simulink model "check_GearSelector"  (R2018b)
settings: configuration reference "Physics" (kept outside this file)
model workspace (MAT data in the model file):
  veh_param = Simulink.Parameter
  veh_param.Value.cLiftF = 0
  veh_param.Value.cLiftR = 0
  veh_param.Value.CoGx_m = 0
  veh_param.Value.CoGy_m = 0
  veh_param.Value.CoGz_m = 0
  veh_param.Value.cDrag = 0
  veh_param.Value.Aref_m2 = 0
  veh_param.Value.Gearratio = 0
  veh_param.Value.Wheelbase_m = 0
  veh_param.Value.PacLatF = [0 0 0 0 0]
  veh_param.Value.PacLongF = [0 0 0 0 0]
  veh_param.Value.PacLatR = [0 0 0 0 0]
  veh_param.Value.PacLongR = [0 0 0 0 0]
  veh_param.Value.cRollFriction_Npmps = 0
  veh_param.Value.MaxRollFriction_N = 0
  veh_param.Value.T_YawRate_s = 0
  veh_param.Value.T_LatVel_s = 0
  veh_param.Value.TrackWidthF_m = 0
  veh_param.Value.TrackWidthR_m = 0
  veh_param.Value.TireRadiusF_m = 0
  veh_param.Value.TireRadiusR_m = 0
  veh_param.Value.VehicleInertia_kgm2 = 0
  veh_param.Value.WheelInertiaF_kgm2 = 0
  veh_param.Value.WheelInertiaR_kgm2 = 0
  veh_param.Value.VehicleMass_kg = 0
  veh_param.Value.switchModelBlend_mps = 0
  veh_param.Value.PTLimitLowVel_N = 0
  veh_param.Value.switchModelVel_mps = 0
  veh_param.Value.T_Tire_s = 0
  veh_param.DataType = 'struct'
  veh_param.Dimensions = [1 1]
  x0_positionstates = Simulink.Parameter
  x0_positionstates.Value = [0 0 0]
  x0_positionstates.DataType = 'auto'
  x0_positionstates.Dimensions = [1 3]
undefined symbols (not defined in the file): POWTR__ENGINE__n_lb_rpm__1, POWTR__ENGINE__n_lb_rpm__2, POWTR__ENGINE__n_lb_rpm__3, POWTR__ENGINE__n_lb_rpm__4, POWTR__ENGINE__n_lb_rpm__5, POWTR__ENGINE__n_lb_rpm__6, POWTR__ENGINE__n_lb_rpm__7, POWTR__ENGINE__n_ub_rpm, POWTR__MODE__activate_ManualGearbox, POWTR__MODE__activate_ThrottleInterface, POWTR__TRANSMISSION__gear__1, POWTR__TRANSMISSION__gear__2, POWTR__TRANSMISSION__gear__3, POWTR__TRANSMISSION__gear__4, POWTR__TRANSMISSION__gear__5, POWTR__TRANSMISSION__gear__6, POWTR__TRANSMISSION__gear__7, POWTR__TRANSMISSION__gear_efficiency__1, POWTR__TRANSMISSION__gear_efficiency__2, POWTR__TRANSMISSION__gear_efficiency__3, POWTR__TRANSMISSION__gear_efficiency__4, POWTR__TRANSMISSION__gear_efficiency__5, POWTR__TRANSMISSION__gear_efficiency__6, POWTR__TRANSMISSION__gear_efficiency__7, POWTR__TRANSMISSION__gear_ratio__1, POWTR__TRANSMISSION__gear_ratio__2, POWTR__TRANSMISSION__gear_ratio__3, POWTR__TRANSMISSION__gear_ratio__4, POWTR__TRANSMISSION__gear_ratio__5, POWTR__TRANSMISSION__gear_ratio__6, POWTR__TRANSMISSION__gear_ratio__7, POWTR__TRANSMISSION__initial_gear
libraries: simulink x2
settings Model: DataDictionary=vehicleparameters_vehdynsim.sldd  OrderedModelArguments=off  Creator=wischnewski  LastModifiedBy=ga25xiw

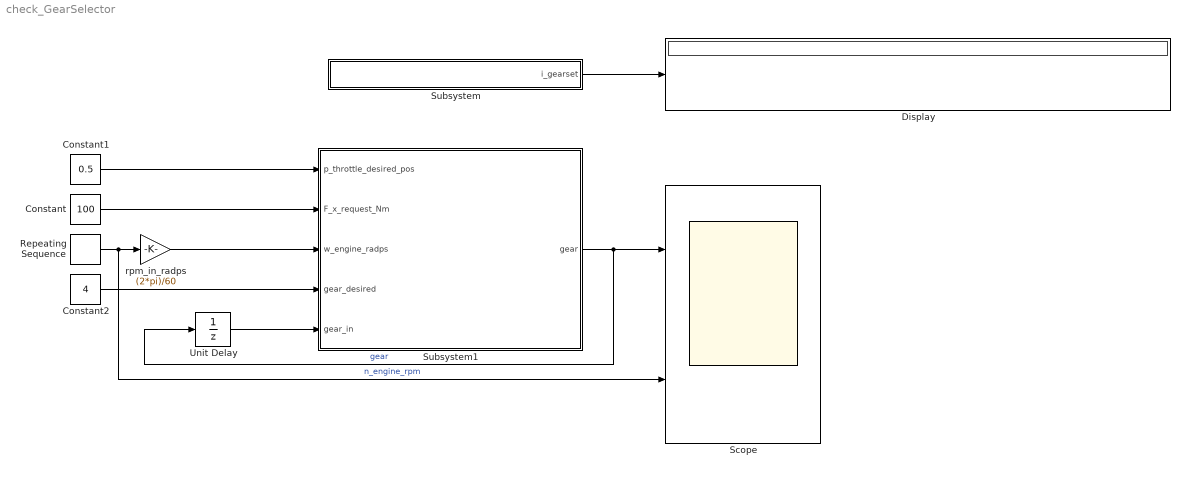
== system check_GearSelector ==
  Constant : Constant  Value=100
  Constant1 : Constant  Value=0.5
  Constant2 : Constant  Value=4
  Display : Display
  Repeating Sequence : simulink/Sources/Repeating Sequence  rep_seq_t=[0 1]  rep_seq_y=[6000 7002]
  Scope : Scope  NumInputPorts=2
  Subsystem : Subsystem
  Subsystem1 : Subsystem
  Unit Delay : UnitDelay  InitialCondition=POWTR__TRANSMISSION__initial_gear  SampleTime=-1
  rpm_in_radps : Gain  Gain=(2*pi)/60
  wires:
  Subsystem/1(i_gearset) -> Display/1
  Subsystem1/1(gear) -> Unit Delay/1, Scope/1  "gear"
  Repeating Sequence/1 -> Scope/2, rpm_in_radps/1  "n_engine_rpm"
  rpm_in_radps/1 -> Subsystem1/3(w_engine_radps)
  Constant/1 -> Subsystem1/2(F_x_request_Nm)
  Constant1/1 -> Subsystem1/1(p_throttle_desired_pos)
  Unit Delay/1 -> Subsystem1/5(gear_in)
  Constant2/1 -> Subsystem1/4(gear_desired)

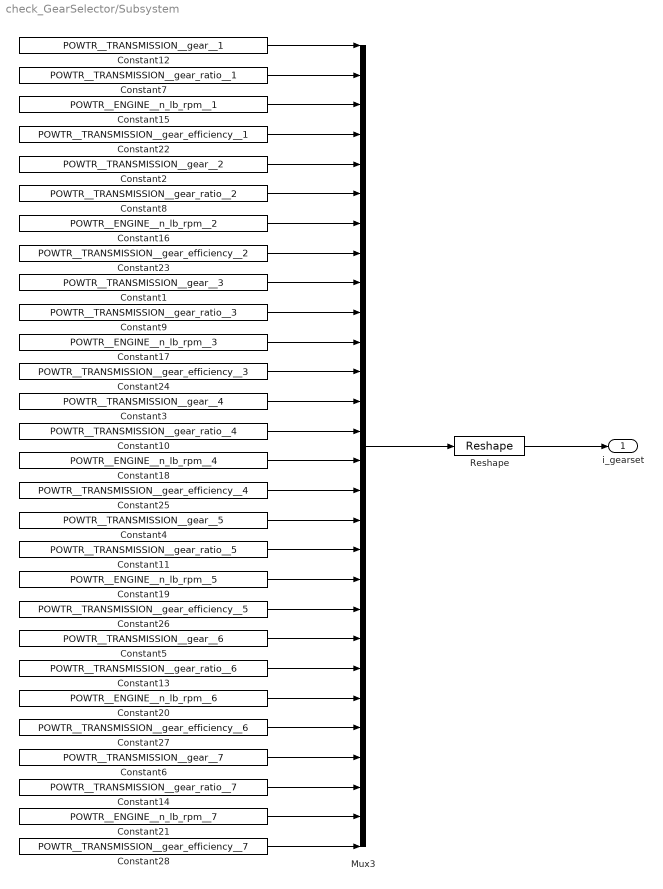
== system check_GearSelector/Subsystem ==
  Constant1 : Constant  Value=POWTR__TRANSMISSION__gear__3
  Constant10 : Constant  Value=POWTR__TRANSMISSION__gear_ratio__4
  Constant11 : Constant  Value=POWTR__TRANSMISSION__gear_ratio__5
  Constant12 : Constant  Value=POWTR__TRANSMISSION__gear__1
  Constant13 : Constant  Value=POWTR__TRANSMISSION__gear_ratio__6
  Constant14 : Constant  Value=POWTR__TRANSMISSION__gear_ratio__7
  Constant15 : Constant  Value=POWTR__ENGINE__n_lb_rpm__1
  Constant16 : Constant  Value=POWTR__ENGINE__n_lb_rpm__2
  Constant17 : Constant  Value=POWTR__ENGINE__n_lb_rpm__3
  Constant18 : Constant  Value=POWTR__ENGINE__n_lb_rpm__4
  Constant19 : Constant  Value=POWTR__ENGINE__n_lb_rpm__5
  Constant2 : Constant  Value=POWTR__TRANSMISSION__gear__2
  Constant20 : Constant  Value=POWTR__ENGINE__n_lb_rpm__6
  Constant21 : Constant  Value=POWTR__ENGINE__n_lb_rpm__7
  Constant22 : Constant  Value=POWTR__TRANSMISSION__gear_efficiency__1
  Constant23 : Constant  Value=POWTR__TRANSMISSION__gear_efficiency__2
  Constant24 : Constant  Value=POWTR__TRANSMISSION__gear_efficiency__3
  Constant25 : Constant  Value=POWTR__TRANSMISSION__gear_efficiency__4
  Constant26 : Constant  Value=POWTR__TRANSMISSION__gear_efficiency__5
  Constant27 : Constant  Value=POWTR__TRANSMISSION__gear_efficiency__6
  Constant28 : Constant  Value=POWTR__TRANSMISSION__gear_efficiency__7
  Constant3 : Constant  Value=POWTR__TRANSMISSION__gear__4
  Constant4 : Constant  Value=POWTR__TRANSMISSION__gear__5
  Constant5 : Constant  Value=POWTR__TRANSMISSION__gear__6
  Constant6 : Constant  Value=POWTR__TRANSMISSION__gear__7
  Constant7 : Constant  Value=POWTR__TRANSMISSION__gear_ratio__1
  Constant8 : Constant  Value=POWTR__TRANSMISSION__gear_ratio__2
  Constant9 : Constant  Value=POWTR__TRANSMISSION__gear_ratio__3
  Mux3 : Mux  Inputs=28
  Reshape : Reshape  OutputDimensionality=Customize  OutputDimensions=[4,7]
  i_gearset : Outport
  wires:
  Mux3/1 -> Reshape/1
  Constant12/1 -> Mux3/1
  Reshape/1 -> i_gearset/1
  Constant2/1 -> Mux3/5
  Constant1/1 -> Mux3/9
  Constant3/1 -> Mux3/13
  Constant4/1 -> Mux3/17
  Constant5/1 -> Mux3/21
  Constant6/1 -> Mux3/25
  Constant7/1 -> Mux3/2
  Constant8/1 -> Mux3/6
  Constant9/1 -> Mux3/10
  Constant10/1 -> Mux3/14
  Constant11/1 -> Mux3/18
  Constant13/1 -> Mux3/22
  Constant14/1 -> Mux3/26
  Constant15/1 -> Mux3/3
  Constant16/1 -> Mux3/7
  Constant17/1 -> Mux3/11
  Constant18/1 -> Mux3/15
  Constant19/1 -> Mux3/19
  Constant20/1 -> Mux3/23
  Constant21/1 -> Mux3/27
  Constant22/1 -> Mux3/4
  Constant23/1 -> Mux3/8
  Constant24/1 -> Mux3/12
  Constant25/1 -> Mux3/16
  Constant26/1 -> Mux3/20
  Constant27/1 -> Mux3/24
  Constant28/1 -> Mux3/28

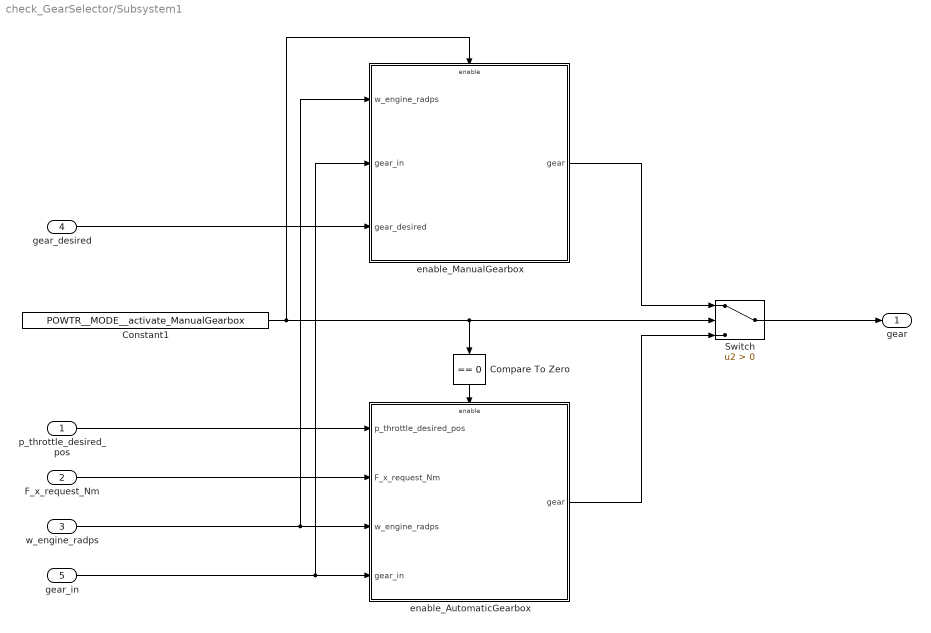
== system check_GearSelector/Subsystem1 ==
  p_throttle_desired_pos : Inport
  F_x_request_Nm : Inport  Port=2
  w_engine_radps : Inport  Port=3
  gear_desired : Inport  Port=4
  gear_in : Inport  Port=5
  Compare To Zero : simulink/Logic and Bit Operations/Compare To Zero  relop===  OutDataTypeStr=boolean
  Constant1 : Constant  Value=POWTR__MODE__activate_ManualGearbox
  Switch : Switch  Criteria=u2 > Threshold
  enable_AutomaticGearbox : Subsystem
  enable_ManualGearbox : Subsystem
  gear : Outport
  wires:
  gear_in/1 -> enable_AutomaticGearbox/4(gear_in), enable_ManualGearbox/2(gear_in)
  gear_desired/1 -> enable_ManualGearbox/3(gear_desired)
  w_engine_radps/1 -> enable_AutomaticGearbox/3(w_engine_radps), enable_ManualGearbox/1(w_engine_radps)
  enable_AutomaticGearbox/1(gear) -> Switch/3
  Compare To Zero/1 -> enable_AutomaticGearbox/Enable
  enable_ManualGearbox/1(gear) -> Switch/1
  p_throttle_desired_pos/1 -> enable_AutomaticGearbox/1(p_throttle_desired_pos)
  Constant1/1 -> Switch/2, Compare To Zero/1, enable_ManualGearbox/Enable
  F_x_request_Nm/1 -> enable_AutomaticGearbox/2(F_x_request_Nm)
  Switch/1 -> gear/1

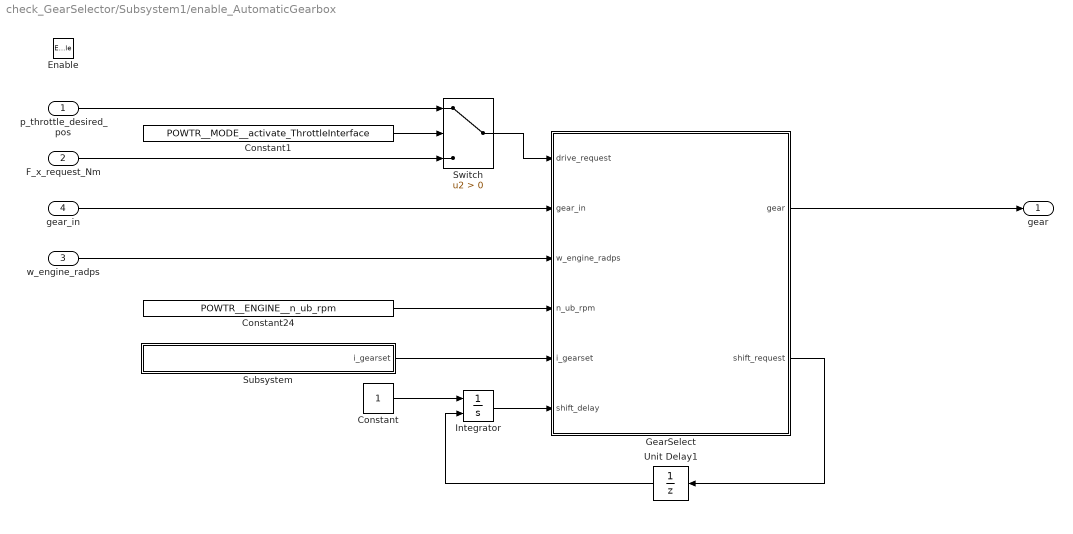
== system check_GearSelector/Subsystem1/enable_AutomaticGearbox ==
  p_throttle_desired_pos : Inport
  F_x_request_Nm : Inport  Port=2
  w_engine_radps : Inport  Port=3
  gear_in : Inport  Port=4
  Enable : EnablePort
  Constant : Constant
  Constant1 : Constant  Value=POWTR__MODE__activate_ThrottleInterface
  Constant24 : Constant  Value=POWTR__ENGINE__n_ub_rpm
  GearSelect : MATLAB Function  TreatAsAtomicUnit=on
  Integrator : Integrator  ExternalReset=rising
  Subsystem : Subsystem
  Switch : Switch  Criteria=u2 > Threshold
  Unit Delay1 : UnitDelay  SampleTime=-1
  gear : Outport
  wires:
  GearSelect/1(gear) -> gear/1
  gear_in/1 -> GearSelect/2(gear_in)
  Constant1/1 -> Switch/2
  Integrator/1 -> GearSelect/6(shift_delay)
  p_throttle_desired_pos/1 -> Switch/1
  w_engine_radps/1 -> GearSelect/3(w_engine_radps)
  Subsystem/1(i_gearset) -> GearSelect/5(i_gearset)
  Unit Delay1/1 -> Integrator/2
  Constant24/1 -> GearSelect/4(n_ub_rpm)
  Constant/1 -> Integrator/1
  Switch/1 -> GearSelect/1(drive_request)
  GearSelect/2(shift_request) -> Unit Delay1/1
  F_x_request_Nm/1 -> Switch/3

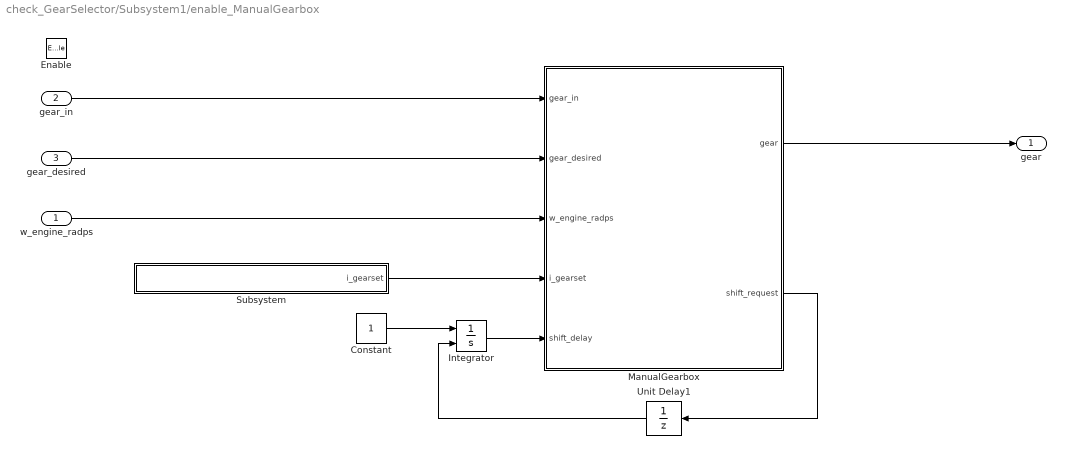
== system check_GearSelector/Subsystem1/enable_ManualGearbox ==
  w_engine_radps : Inport
  gear_in : Inport  Port=2
  gear_desired : Inport  Port=3
  Enable : EnablePort
  Constant : Constant
  Integrator : Integrator  ExternalReset=rising
  ManualGearbox : MATLAB Function  TreatAsAtomicUnit=on
  Subsystem : Subsystem
  Unit Delay1 : UnitDelay  SampleTime=-1
  gear : Outport
  wires:
  ManualGearbox/2(shift_request) -> Unit Delay1/1
  Constant/1 -> Integrator/1
  Unit Delay1/1 -> Integrator/2
  Subsystem/1(i_gearset) -> ManualGearbox/4(i_gearset)
  w_engine_radps/1 -> ManualGearbox/3(w_engine_radps)
  Integrator/1 -> ManualGearbox/5(shift_delay)
  gear_in/1 -> ManualGearbox/1(gear_in)
  ManualGearbox/1(gear) -> gear/1
  gear_desired/1 -> ManualGearbox/2(gear_desired)

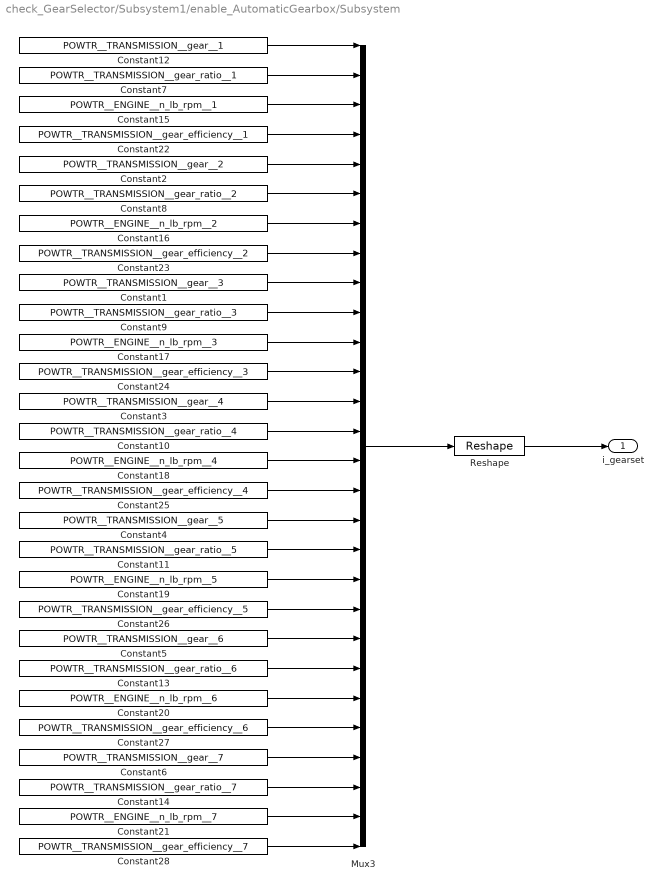
== system check_GearSelector/Subsystem1/enable_AutomaticGearbox/Subsystem ==
  Constant1 : Constant  Value=POWTR__TRANSMISSION__gear__3
  Constant10 : Constant  Value=POWTR__TRANSMISSION__gear_ratio__4
  Constant11 : Constant  Value=POWTR__TRANSMISSION__gear_ratio__5
  Constant12 : Constant  Value=POWTR__TRANSMISSION__gear__1
  Constant13 : Constant  Value=POWTR__TRANSMISSION__gear_ratio__6
  Constant14 : Constant  Value=POWTR__TRANSMISSION__gear_ratio__7
  Constant15 : Constant  Value=POWTR__ENGINE__n_lb_rpm__1
  Constant16 : Constant  Value=POWTR__ENGINE__n_lb_rpm__2
  Constant17 : Constant  Value=POWTR__ENGINE__n_lb_rpm__3
  Constant18 : Constant  Value=POWTR__ENGINE__n_lb_rpm__4
  Constant19 : Constant  Value=POWTR__ENGINE__n_lb_rpm__5
  Constant2 : Constant  Value=POWTR__TRANSMISSION__gear__2
  Constant20 : Constant  Value=POWTR__ENGINE__n_lb_rpm__6
  Constant21 : Constant  Value=POWTR__ENGINE__n_lb_rpm__7
  Constant22 : Constant  Value=POWTR__TRANSMISSION__gear_efficiency__1
  Constant23 : Constant  Value=POWTR__TRANSMISSION__gear_efficiency__2
  Constant24 : Constant  Value=POWTR__TRANSMISSION__gear_efficiency__3
  Constant25 : Constant  Value=POWTR__TRANSMISSION__gear_efficiency__4
  Constant26 : Constant  Value=POWTR__TRANSMISSION__gear_efficiency__5
  Constant27 : Constant  Value=POWTR__TRANSMISSION__gear_efficiency__6
  Constant28 : Constant  Value=POWTR__TRANSMISSION__gear_efficiency__7
  Constant3 : Constant  Value=POWTR__TRANSMISSION__gear__4
  Constant4 : Constant  Value=POWTR__TRANSMISSION__gear__5
  Constant5 : Constant  Value=POWTR__TRANSMISSION__gear__6
  Constant6 : Constant  Value=POWTR__TRANSMISSION__gear__7
  Constant7 : Constant  Value=POWTR__TRANSMISSION__gear_ratio__1
  Constant8 : Constant  Value=POWTR__TRANSMISSION__gear_ratio__2
  Constant9 : Constant  Value=POWTR__TRANSMISSION__gear_ratio__3
  Mux3 : Mux  Inputs=28
  Reshape : Reshape  OutputDimensionality=Customize  OutputDimensions=[4,7]
  i_gearset : Outport
  wires:
  Mux3/1 -> Reshape/1
  Constant12/1 -> Mux3/1
  Reshape/1 -> i_gearset/1
  Constant2/1 -> Mux3/5
  Constant1/1 -> Mux3/9
  Constant3/1 -> Mux3/13
  Constant4/1 -> Mux3/17
  Constant5/1 -> Mux3/21
  Constant6/1 -> Mux3/25
  Constant7/1 -> Mux3/2
  Constant8/1 -> Mux3/6
  Constant9/1 -> Mux3/10
  Constant10/1 -> Mux3/14
  Constant11/1 -> Mux3/18
  Constant13/1 -> Mux3/22
  Constant14/1 -> Mux3/26
  Constant15/1 -> Mux3/3
  Constant16/1 -> Mux3/7
  Constant17/1 -> Mux3/11
  Constant18/1 -> Mux3/15
  Constant19/1 -> Mux3/19
  Constant20/1 -> Mux3/23
  Constant21/1 -> Mux3/27
  Constant22/1 -> Mux3/4
  Constant23/1 -> Mux3/8
  Constant24/1 -> Mux3/12
  Constant25/1 -> Mux3/16
  Constant26/1 -> Mux3/20
  Constant27/1 -> Mux3/24
  Constant28/1 -> Mux3/28

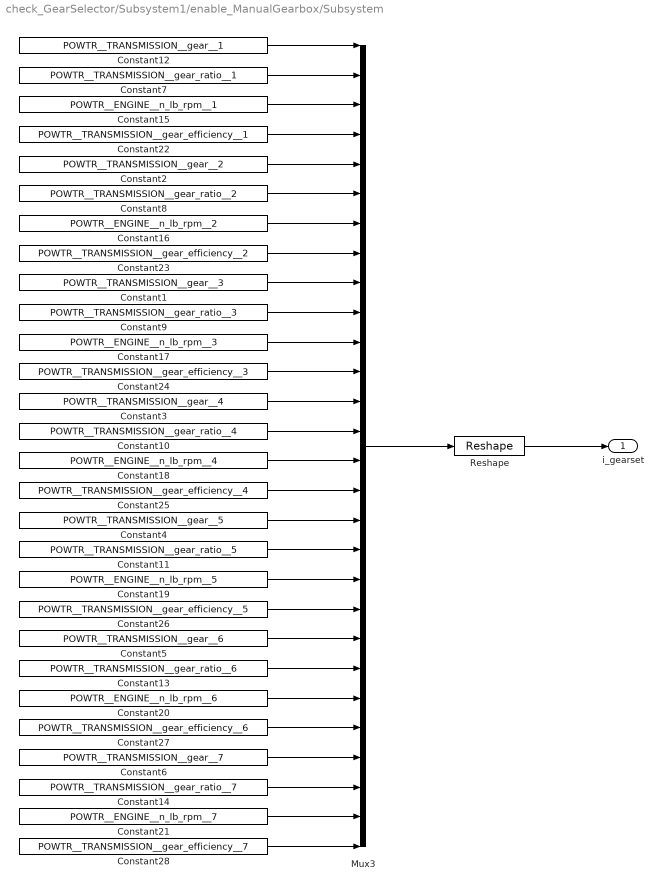
== system check_GearSelector/Subsystem1/enable_ManualGearbox/Subsystem ==
  Constant1 : Constant  Value=POWTR__TRANSMISSION__gear__3
  Constant10 : Constant  Value=POWTR__TRANSMISSION__gear_ratio__4
  Constant11 : Constant  Value=POWTR__TRANSMISSION__gear_ratio__5
  Constant12 : Constant  Value=POWTR__TRANSMISSION__gear__1
  Constant13 : Constant  Value=POWTR__TRANSMISSION__gear_ratio__6
  Constant14 : Constant  Value=POWTR__TRANSMISSION__gear_ratio__7
  Constant15 : Constant  Value=POWTR__ENGINE__n_lb_rpm__1
  Constant16 : Constant  Value=POWTR__ENGINE__n_lb_rpm__2
  Constant17 : Constant  Value=POWTR__ENGINE__n_lb_rpm__3
  Constant18 : Constant  Value=POWTR__ENGINE__n_lb_rpm__4
  Constant19 : Constant  Value=POWTR__ENGINE__n_lb_rpm__5
  Constant2 : Constant  Value=POWTR__TRANSMISSION__gear__2
  Constant20 : Constant  Value=POWTR__ENGINE__n_lb_rpm__6
  Constant21 : Constant  Value=POWTR__ENGINE__n_lb_rpm__7
  Constant22 : Constant  Value=POWTR__TRANSMISSION__gear_efficiency__1
  Constant23 : Constant  Value=POWTR__TRANSMISSION__gear_efficiency__2
  Constant24 : Constant  Value=POWTR__TRANSMISSION__gear_efficiency__3
  Constant25 : Constant  Value=POWTR__TRANSMISSION__gear_efficiency__4
  Constant26 : Constant  Value=POWTR__TRANSMISSION__gear_efficiency__5
  Constant27 : Constant  Value=POWTR__TRANSMISSION__gear_efficiency__6
  Constant28 : Constant  Value=POWTR__TRANSMISSION__gear_efficiency__7
  Constant3 : Constant  Value=POWTR__TRANSMISSION__gear__4
  Constant4 : Constant  Value=POWTR__TRANSMISSION__gear__5
  Constant5 : Constant  Value=POWTR__TRANSMISSION__gear__6
  Constant6 : Constant  Value=POWTR__TRANSMISSION__gear__7
  Constant7 : Constant  Value=POWTR__TRANSMISSION__gear_ratio__1
  Constant8 : Constant  Value=POWTR__TRANSMISSION__gear_ratio__2
  Constant9 : Constant  Value=POWTR__TRANSMISSION__gear_ratio__3
  Mux3 : Mux  Inputs=28
  Reshape : Reshape  OutputDimensionality=Customize  OutputDimensions=[4,7]
  i_gearset : Outport
  wires:
  Constant28/1 -> Mux3/28
  Constant27/1 -> Mux3/24
  Constant26/1 -> Mux3/20
  Constant25/1 -> Mux3/16
  Constant24/1 -> Mux3/12
  Constant23/1 -> Mux3/8
  Constant22/1 -> Mux3/4
  Constant21/1 -> Mux3/27
  Constant20/1 -> Mux3/23
  Constant19/1 -> Mux3/19
  Constant18/1 -> Mux3/15
  Constant17/1 -> Mux3/11
  Constant16/1 -> Mux3/7
  Constant15/1 -> Mux3/3
  Constant14/1 -> Mux3/26
  Constant13/1 -> Mux3/22
  Constant11/1 -> Mux3/18
  Constant10/1 -> Mux3/14
  Constant9/1 -> Mux3/10
  Constant8/1 -> Mux3/6
  Constant7/1 -> Mux3/2
  Constant6/1 -> Mux3/25
  Constant5/1 -> Mux3/21
  Constant4/1 -> Mux3/17
  Constant3/1 -> Mux3/13
  Constant1/1 -> Mux3/9
  Constant2/1 -> Mux3/5
  Reshape/1 -> i_gearset/1
  Constant12/1 -> Mux3/1
  Mux3/1 -> Reshape/1

== matlab function check_GearSelector/Subsystem1/enable_ManualGearbox/ManualGearbox ==
  data: gear_in input; gear_desired input; gear output; w_engine_radps input; i_gearset input; shift_delay input; shift_request output
function [gear, shift_request] = fcn(gear_in, gear_desired, ...
                            w_engine_radps, i_gearset, shift_delay)

[gear, shift_request] = ManualGearbox(gear_in, gear_desired, ...
                            w_engine_radps, i_gearset, shift_delay);

== matlab function check_GearSelector/Subsystem1/enable_AutomaticGearbox/GearSelect ==
  data: drive_request input; gear_in input; gear output; w_engine_radps input; n_ub_rpm input; i_gearset input; shift_delay input; shift_request output
function [gear, shift_request] = fcn(drive_request, gear_in, ...
                            w_engine_radps, n_ub_rpm, i_gearset, shift_delay)

[gear, shift_request] = AutomaticGearbox(drive_request, gear_in, ...
                            w_engine_radps, n_ub_rpm, i_gearset, shift_delay);
